simulink subsystem "Throttle_Map_2WD_NO_REGEN"  (R2023b)
settings: Solver=VariableStepAuto  StartTime=0.0  StopTime=10.0  RelTol=1e-3
undefined symbols (not defined in the file or in its folder): alpha, dK, dk_thresh, FINISHED_SMOOTHENING_IC, k_IC, LAST_TVS_PERMIT_IC, minK, V, w
settings Model: Creator=Inver  LastModifiedBy=Inver

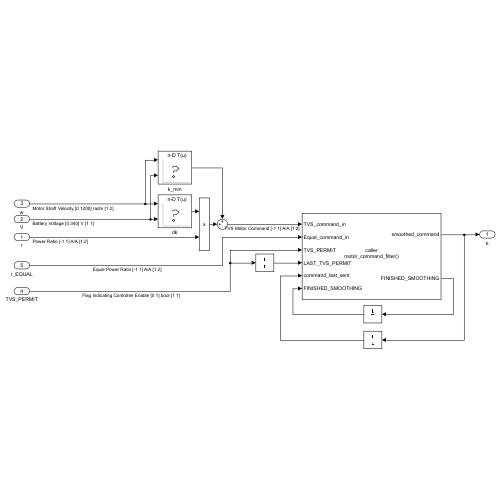
[thumbnail: Simulink's stored preview of the top-level diagram]
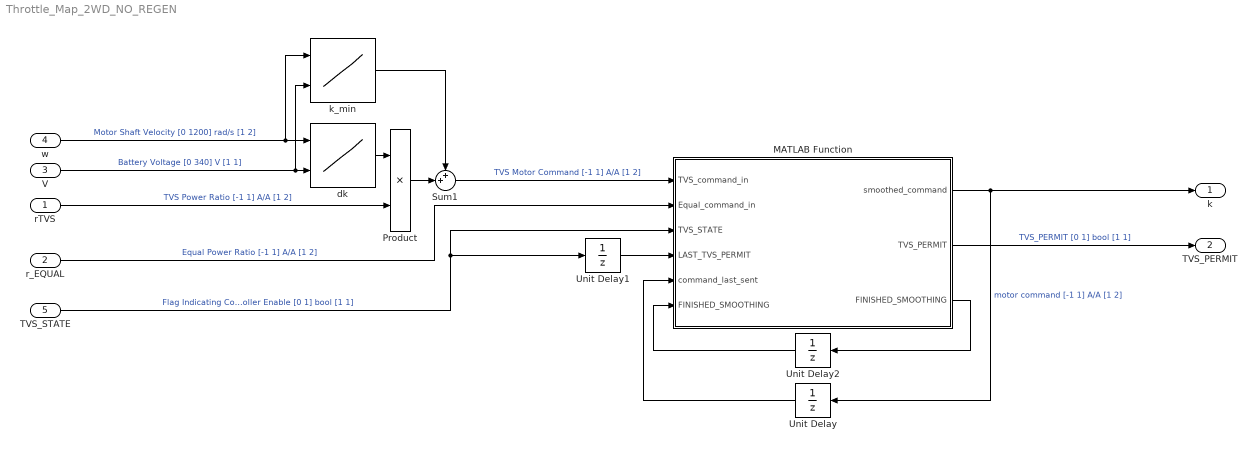
== system Throttle_Map_2WD_NO_REGEN ==
  rTVS : Inport
  r_EQUAL : Inport  Port=2
  V : Inport  Port=3
  w : Inport  Port=4
  TVS_STATE : Inport  Port=5
  MATLAB Function : MATLAB Function  TreatAsAtomicUnit=on
  Product : Product
  Sum1 : Sum  Inputs=++|
  Unit Delay : UnitDelay  InitialCondition=k_IC  SampleTime=-1  HasFrameUpgradeWarning=on
  Unit Delay1 : UnitDelay  InitialCondition=LAST_TVS_PERMIT_IC  SampleTime=-1  HasFrameUpgradeWarning=on
  Unit Delay2 : UnitDelay  InitialCondition=FINISHED_SMOOTHENING_IC  SampleTime=-1  HasFrameUpgradeWarning=on
  dk : Lookup_n-D  LookupTableObject=''  BreakpointsForDimension1=w  BreakpointsForDimension2=V  BreakpointsForDimension1FirstPoint=10  BreakpointsForDimension2FirstPoint=10  BreakpointsForDimension1Spacing=12  BreakpointsForDimension2Spacing=12  IndexSearchMethod=Evenly spaced points  BeginIndexSearchUsingPreviousIndexResult=on  Table=dK  ExtrapMethod=Clip  DiagnosticForOutOfRangeInput=Error  RemoveProtectionInput=on  UseLastTableValue=on  InternalRulePriority=Speed  RndMeth=Simplest
      settings: InputPortMap=u0,u1
  k_min : Lookup_n-D  LookupTableObject=''  BreakpointsForDimension1=w  BreakpointsForDimension2=V  BreakpointsForDimension1FirstPoint=10  BreakpointsForDimension2FirstPoint=10  BreakpointsForDimension1Spacing=12  BreakpointsForDimension2Spacing=12  IndexSearchMethod=Evenly spaced points  BeginIndexSearchUsingPreviousIndexResult=on  Table=minK  ExtrapMethod=Clip  DiagnosticForOutOfRangeInput=Error  RemoveProtectionInput=on  UseLastTableValue=on  InternalRulePriority=Speed  RndMeth=Simplest
      settings: InputPortMap=u0,u1
  k : Outport
  TVS_PERMIT : Outport  Port=2
  wires:
  w/1 -> dk/1, k_min/1  "Motor Shaft Velocity [0 1200] rad/s [1 2]"
  V/1 -> dk/2, k_min/2  "Battery Voltage [0 340] V [1 1]"
  rTVS/1 -> Product/2  "TVS Power Ratio [-1 1] A/A [1 2]"
  Sum1/1 -> MATLAB Function/1(TVS_command_in)  "TVS Motor Command [-1 1] A/A [1 2]"
  k_min/1 -> Sum1/1
  dk/1 -> Product/1
  Product/1 -> Sum1/2
  TVS_STATE/1 -> MATLAB Function/3(TVS_STATE), Unit Delay1/1  "Flag Indicating Controller Enable [0 1] bool [1 1]"
  r_EQUAL/1 -> MATLAB Function/2(Equal_command_in)  "Equal Power Ratio [-1 1] A/A [1 2]"
  MATLAB Function/1(smoothed_command) -> k/1, Unit Delay/1  "motor command [-1 1] A/A [1 2]"
  Unit Delay/1 -> MATLAB Function/5(command_last_sent)
  MATLAB Function/3(FINISHED_SMOOTHING) -> Unit Delay2/1
  Unit Delay2/1 -> MATLAB Function/6("FINISHED_SMOOTHING ")
  Unit Delay1/1 -> MATLAB Function/4(LAST_TVS_PERMIT)
  MATLAB Function/2(TVS_PERMIT) -> TVS_PERMIT/1  "TVS_PERMIT [0 1] bool [1 1]"

== matlab function Throttle_Map_2WD_NO_REGEN/MATLAB Function ==
  data: TVS_command_in input size=[ 1 2]; smoothed_command output size=[1 2]; TVS_PERMIT output; Equal_command_in input size=[1 2]; TVS_STATE input; LAST_TVS_PERMIT input; command_last_sent input size=[1 2]; FINISHED_SMOOTHING input; FINISHED_SMOOTHING output; alpha parameter; dk_thresh parameter
function [smoothed_command, TVS_PERMIT, FINISHED_SMOOTHING] = motor_command_filter(TVS_command_in, Equal_command_in, TVS_STATE, LAST_TVS_PERMIT, command_last_sent, FINISHED_SMOOTHING,alpha,dk_thresh)
% Filters motor comands during TVS mode changes
%   Detailed explanation goes here
smoothed_command = zeros(1,2);

% switch between modes
if TVS_STATE
    command_in = TVS_command_in;
else
    command_in = Equal_command_in;
end

if TVS_STATE ~= LAST_TVS_PERMIT % TVS changed
    FINISHED_SMOOTHING = 0;
end

if command_last_sent(1) > command_last_sent(2)
    low_command = command_last_sent(2);
    low_dif = min(command_in) - low_command;

    if abs(low_dif) < dk_thresh % signals are close enough
        FINISHED_SMOOTHING = 1;
    end

    if FINISHED_SMOOTHING == 0 % continue smoothing
        filt_dif = alpha * low_dif + (1-alpha) * 0;
        smoothed_command(2) = min(low_command + filt_dif, max(command_in));
        smoothed_command(1) = max(command_in);
    else
        smoothed_command = command_in;
    end
else
    low_command = command_last_sent(1);
    low_dif = min(command_in) - low_command;

    if abs(low_dif) < dk_thresh % signals are close enough
        FINISHED_SMOOTHING = 1;
    end

    if FINISHED_SMOOTHING == 0 % continue smoothing
        filt_dif = alpha * low_dif + (1-alpha) * 0;
        smoothed_command(1) = min(low_command + filt_dif, max(command_in));
        smoothed_command(2) = max(command_in);
    else
        smoothed_command = command_in;
    end
end

if FINISHED_SMOOTHING && (~TVS_STATE)
    TVS_PERMIT = 0;
else
    TVS_PERMIT = 1;
end
